simulink model "Terceira_lei_de_controle"  (R2015b)
settings: Solver=VariableStepAuto  StartTime=0.0  StopTime=10.0  RelTol=1e-3
settings Model: Creator=egidio.neto  LastModifiedBy=egidio.neto

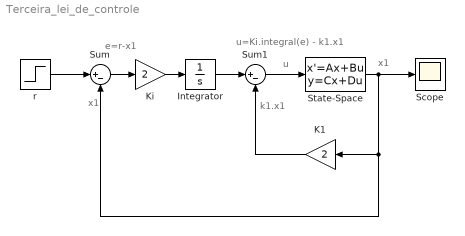
== system Terceira_lei_de_controle ==
  note: k1.x1
  note: u
  note: e=r-x1
  note: x1
  note: x1
  note: u=Ki.integral(e) - k1.x1
  Integrator : Integrator
  K1 : Gain  Gain=2
  Ki : Gain  Gain=2
  Scope : Scope
  State-Space : StateSpace  A=[1]  B=[1]  C=[1]  D=[0]  X0=[0]
  Sum : Sum  Inputs=|+-
  Sum1 : Sum  Inputs=|+-
  r : Step  SampleTime=0
  wires:
  r/1 -> Sum/1
  Sum/1 -> Ki/1
  K1/1 -> Sum1/2
  Sum1/1 -> State-Space/1
  State-Space/1 -> Scope/1, K1/1, Sum/2
  Ki/1 -> Integrator/1
  Integrator/1 -> Sum1/1
